simulink model "Sistema"  (R2024b)
settings: Solver=ode15s  StartTime=0.0  StopTime=10.0  MaxStep=1e-3  RelTol=1e-3
libraries: slpidlib x1
settings Model: Creator=Lenovo
settings DataIOCC: ReturnWorkspaceOutputs=off  TimeSaveName=t
settings DebuggingCC: AlgebraicLoopMsg=none  ArtificialAlgebraicLoopMsg=none
settings RTWCC: GPUComputeCapability=3.5

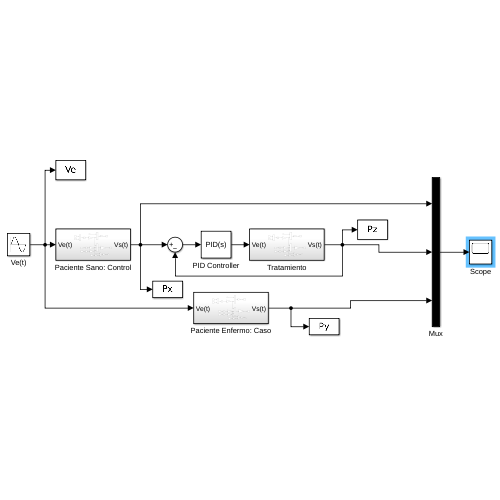
[thumbnail: Simulink's stored preview of the top-level diagram]
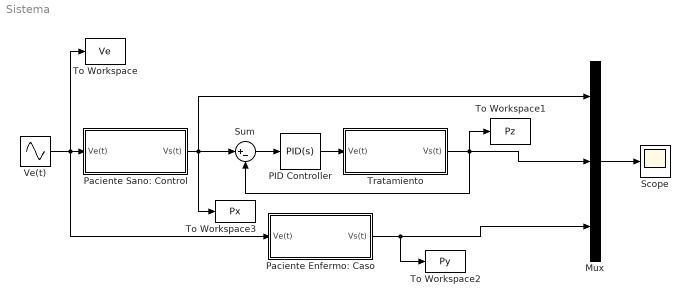
== system Sistema ==
  Mux : Mux  Inputs=3
  PID Controller : slpidlib/PID Controller  Controller=PID  Form=Parallel  TimeDomain=Continuous-time  UseExternalTs=off  SampleTime=-1  IntegratorMethod=Forward Euler  FilterMethod=Forward Euler  ControllerParametersSource=internal  P=161.804025954698  I=4037.58496324393  UseKiTs=off  D=0.223991243195412  UseExternalDerivativeSource=off  N=515.816699684725  UseFilter=on  TunerSelectOption=Transfer Function Based (PID Tuner App)  InitialConditionSource=internal  InitialConditionForIntegrator=0  InitialConditionForFilter=0  DifferentiatorICPrevScaledInput=0  ExternalReset=none  TrackingMode=off  Kt=1  LimitOutput=off  SatLimitsSource=internal  UpperSaturationLimit=inf  LowerSaturationLimit=-inf  LinearizeAsGain=on  AntiWindupMode=none  Kb=1  LimitIntegrator=off  UpperIntegratorSaturationLimit=inf  LowerIntegratorSaturationLimit=-inf  POutMin=[]  POutMax=[]  IOutMin=[]  IOutMax=[]  DOutMin=[]  DOutMax=[]  NOutMin=[]  NOutMax=[]  SumOutMin=[]  SumOutMax=[]  SaturationOutMin=[]  SaturationOutMax=[]  PParamMin=[]  PParamMax=[]  IParamMin=[]  IParamMax=[]  DParamMin=[]  DParamMax=[]  NParamMin=[]  NParamMax=[]  KbParamMin=[]  KbParamMax=[]  KtParamMin=[]  KtParamMax=[]  KbOutMin=[]  KbOutMax=[]  KtOutMin=[]  KtOutMax=[]  IntegratorOutMin=[]  IntegratorOutMax=[]  FilterOutMin=[]  FilterOutMax=[]  SumI1OutMin=[]  SumI1OutMax=[]  SumI2OutMin=[]  SumI2OutMax=[]  SumI3OutMin=[]  SumI3OutMax=[]  SumI4OutMin=[]  SumI4OutMax=[]  SumDOutMin=[]  SumDOutMax=[]  DifferentiatorOutMin=[]  DifferentiatorOutMax=[]  FilterDiffOutCoefMin=[]  FilterDiffOutCoefMax=[]  ReciprocalOutMin=[]  ReciprocalOutMax=[]  SumDenOutMin=[]  SumDenOutMax=[]  SumNumOutMin=[]  SumNumOutMax=[]  DivideOutMin=[]  DivideOutMax=[]  UdiffTsProdOutMin=[]  UdiffTsProdOutMax=[]  NTsProdOutMin=[]  NTsProdOutMax=[]  UintegralTsProdOutMin=[]  UintegralTsProdOutMax=[]  UngainTsProdOutMin=[]  UngainTsProdOutMax=[]  ClampingZeroOutDataTypeStr=Inherit: Inherit via back propagation  ClampingZeroOutMin=[]  ClampingZeroOutMax=[]  FilterDenConstantOutDataTypeStr=Inherit: Inherit via back propagation  FilterDenConstantOutMin=[]  FilterDenConstantOutMax=[]  PCopyOutDataTypeStr=Inherit: Inherit via back propagation  PCopyOutMin=[]  PCopyOutMax=[]  NCopyOutDataTypeStr=Inherit: Inherit via back propagation  NCopyOutMin=[]  NCopyOutMax=[]  IntegratorContinuousStateAttributes=''  IntegratorStateMustResolveToSignalObject=off  IntegratorRTWStateStorageClass=Auto  FilterContinuousStateAttributes=''  FilterStateMustResolveToSignalObject=off  FilterRTWStateStorageClass=Auto  ParallelPVariant=InternalParameters  IdealPVariant=Disabled  IVariant=InternalParameters  DVariant=InternalParameters  IntegratorVariant=Continuous  SatVariant=Disabled  AWVariant=Passthrough  PCopyVariant=Disabled  TRVariant=Disabled  FdbkBlocksVariant=Forward  IdealPFdbkVariant=Disabled  SatFdbkVariant=Disabled  DerivativeFilterVariant=ContFilter  NVariant=InternalParameters  NCopyVariant=Disabled  FilterICVariant=InternalICsFilter  IntegratorICVariant=InternalICs  ExternalResetVariant=Disabled  TRSumVariant=Passthrough  SumFdbkVariant=Disabled  SumVariant=Sum_PID  TsampFilterVariant=InternalTs  TsampNgainVariant=Passthrough  TsampIntegralVariant=Disabled_SignalSpec  ExternalSaturationOutDataTypeStr=Inherit: Same as second input  DerivativeSourceVariant=ErrorSignal  PreIntVariant=InternalPreInt
  Paciente Enfermo: Caso : Subsystem
  Paciente Sano: Control : Subsystem
  Scope : Scope
  Sum : Sum  Inputs=|+-
  To Workspace : ToWorkspace  VariableName=Ve  SampleTime=-1
  To Workspace1 : ToWorkspace  VariableName=Pz  SampleTime=-1
  To Workspace2 : ToWorkspace  VariableName=Py  SampleTime=-1
  To Workspace3 : ToWorkspace  VariableName=Px  SampleTime=-1
  Tratamiento : Subsystem
  Ve(t) : Sin  Frequency=2*pi  SampleTime=0
  wires:
  Mux/1 -> Scope/1
  Sum/1 -> PID Controller/1
  Paciente Sano: Control/1(Vs(t)) -> Mux/1, To Workspace3/1, Sum/1
  Ve(t)/1 -> Paciente Enfermo: Caso/1(Ve(t)), Paciente Sano: Control/1(Ve(t)), To Workspace/1
  Paciente Enfermo: Caso/1(Vs(t)) -> To Workspace2/1, Mux/3
  PID Controller/1 -> Tratamiento/1(Ve(t))
  Tratamiento/1(Vs(t)) -> To Workspace1/1, Sum/2, Mux/2

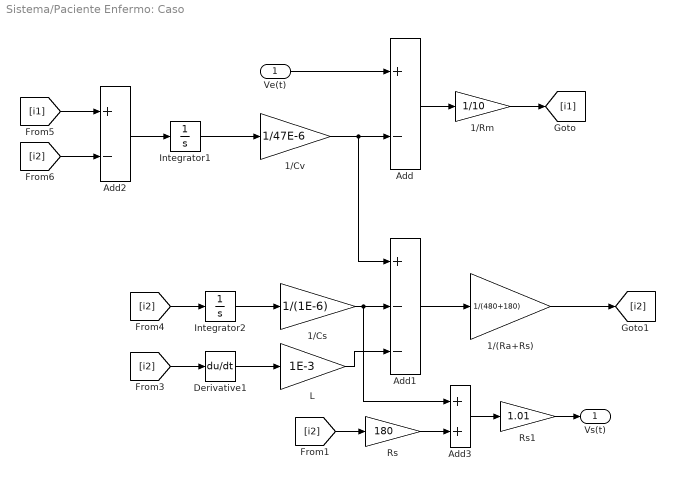
== system Sistema/Paciente Enfermo: Caso ==
  Ve(t) : Inport
  1/(Ra+Rs) : Gain  Gain=1/(480+180)
  1/Cs : Gain  Gain=1/(1E-6)
  1/Cv : Gain  Gain=1/47E-6
  1/Rm : Gain  Gain=1/10
  Add : Sum  Inputs=+-
  Add1 : Sum  Inputs=+--
  Add2 : Sum  Inputs=+-
  Add3 : Sum
  Derivative1 : Derivative
  Integrator1 : Integrator
  Integrator2 : Integrator
  L : Gain  Gain=1E-3
  Rs : Gain  Gain=180
  Rs1 : Gain  Gain=1.01
  Vs(t) : Outport
  wires:
  Integrator2/1 -> 1/Cs/1
  Add1/1 -> 1/(Ra+Rs)/1
  Integrator1/1 -> 1/Cv/1
  1/Cv/1 -> Add1/1, Add/2
  Add/1 -> 1/Rm/1
  Ve(t)/1 -> Add/1
  L/1 -> Add1/3
  Add3/1 -> Rs1/1
  1/(Ra+Rs)/1 -> [i2]
  [i2] -> Rs/1
  Derivative1/1 -> L/1
  [i2] -> Integrator2/1
  Rs/1 -> Add3/2
  [i2] -> Derivative1/1
  1/Rm/1 -> [i1]
  [i1] -> Add2/1
  1/Cs/1 -> Add1/2, Add3/1
  [i2] -> Add2/2
  Add2/1 -> Integrator1/1
  Rs1/1 -> Vs(t)/1

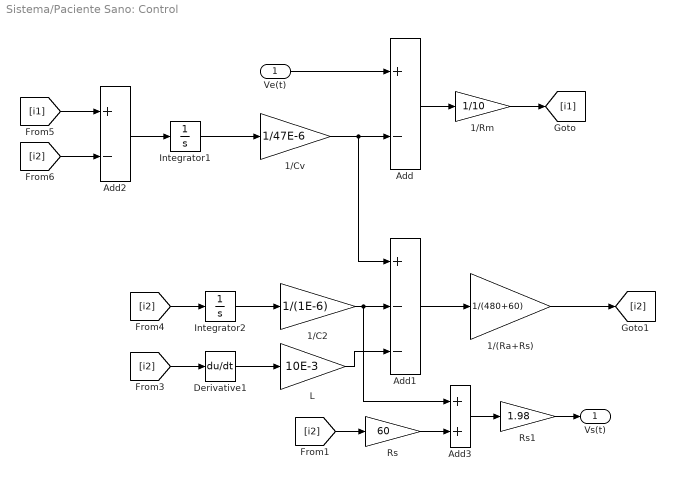
== system Sistema/Paciente Sano: Control ==
  Ve(t) : Inport
  1/(Ra+Rs) : Gain  Gain=1/(480+60)
  1/C2 : Gain  Gain=1/(1E-6)
  1/Cv : Gain  Gain=1/47E-6
  1/Rm : Gain  Gain=1/10
  Add : Sum  Inputs=+-
  Add1 : Sum  Inputs=+--
  Add2 : Sum  Inputs=+-
  Add3 : Sum
  Derivative1 : Derivative
  Integrator1 : Integrator
  Integrator2 : Integrator
  L : Gain  Gain=10E-3
  Rs : Gain  Gain=60
  Rs1 : Gain  Gain=1.98
  Vs(t) : Outport
  wires:
  [i2] -> Add2/2
  [i1] -> Add2/1
  1/Cv/1 -> Add1/1, Add/2
  1/Rm/1 -> [i1]
  Add1/1 -> 1/(Ra+Rs)/1
  Integrator1/1 -> 1/Cv/1
  Add2/1 -> Integrator1/1
  Add/1 -> 1/Rm/1
  Ve(t)/1 -> Add/1
  1/(Ra+Rs)/1 -> [i2]
  1/C2/1 -> Add1/2, Add3/1
  L/1 -> Add1/3
  Derivative1/1 -> L/1
  [i2] -> Derivative1/1
  [i2] -> Integrator2/1
  Integrator2/1 -> 1/C2/1
  Add3/1 -> Rs1/1
  Rs/1 -> Add3/2
  [i2] -> Rs/1
  Rs1/1 -> Vs(t)/1

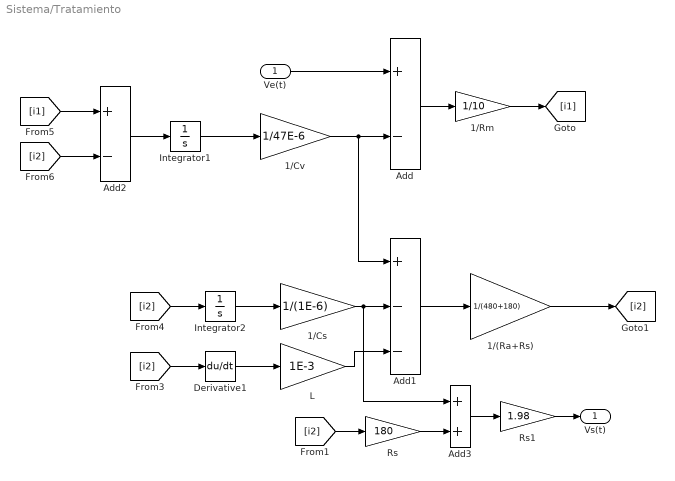
== system Sistema/Tratamiento ==
  Ve(t) : Inport
  1/(Ra+Rs) : Gain  Gain=1/(480+180)
  1/Cs : Gain  Gain=1/(1E-6)
  1/Cv : Gain  Gain=1/47E-6
  1/Rm : Gain  Gain=1/10
  Add : Sum  Inputs=+-
  Add1 : Sum  Inputs=+--
  Add2 : Sum  Inputs=+-
  Add3 : Sum
  Derivative1 : Derivative
  Integrator1 : Integrator
  Integrator2 : Integrator
  L : Gain  Gain=1E-3
  Rs : Gain  Gain=180
  Rs1 : Gain  Gain=1.98
  Vs(t) : Outport
  wires:
  Integrator2/1 -> 1/Cs/1
  Rs/1 -> Add3/2
  1/Cv/1 -> Add1/1, Add/2
  Integrator1/1 -> 1/Cv/1
  Derivative1/1 -> L/1
  Ve(t)/1 -> Add/1
  Add1/1 -> 1/(Ra+Rs)/1
  L/1 -> Add1/3
  [i2] -> Add2/2
  1/(Ra+Rs)/1 -> [i2]
  Add/1 -> 1/Rm/1
  [i1] -> Add2/1
  Add2/1 -> Integrator1/1
  1/Rm/1 -> [i1]
  [i2] -> Integrator2/1
  [i2] -> Derivative1/1
  Add3/1 -> Rs1/1
  1/Cs/1 -> Add1/2, Add3/1
  [i2] -> Rs/1
  Rs1/1 -> Vs(t)/1
